simulink model "test_libMdl_Imu"  (R2018a)
settings: Solver=FixedStepAuto  StartTime=0.0  StopTime=50  RelTol=1e-3
libraries: simulink x2, libMdl_Imu x1
settings Model: Creator=hwinter  LastModifiedBy=hwinter

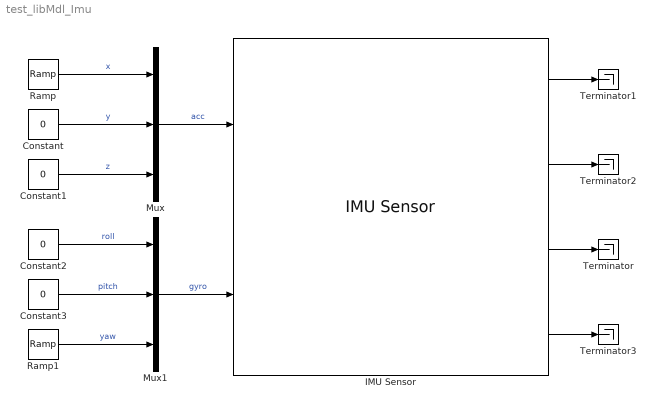
== system test_libMdl_Imu ==
  Constant{,1..3} (4 alike) : Constant  Value=0
  IMU Sensor : libMdl_Imu/IMU Sensor  mv_T_imu=1  mv_sigma_imu_acc=[1 1 1]  mv_sigma_imu_gyro=[1 1 1]  mv_z_0_imu_acc=[0 0 0]  mv_z_0_imu_gyro=[0 0 0]  mv_seed_imu=71322
  Mux : Mux  Inputs=3
  Mux1 : Mux  Inputs=3
  Ramp : simulink/Sources/Ramp  slope=1  start=0  InitialOutput=0
  Ramp1 : simulink/Sources/Ramp  slope=1  start=0  InitialOutput=0
  Terminator{,1..3} (4 alike) : Terminator
  wires:
  Constant/1 -> Mux/2  "y"
  Mux/1 -> IMU Sensor/1  "acc"
  IMU Sensor/3 -> Terminator/1
  IMU Sensor/1 -> Terminator1/1
  Constant1/1 -> Mux/3  "z"
  Mux1/1 -> IMU Sensor/2  "gyro"
  Constant3/1 -> Mux1/2  "pitch"
  Constant2/1 -> Mux1/1  "roll"
  IMU Sensor/4 -> Terminator3/1
  IMU Sensor/2 -> Terminator2/1
  Ramp1/1 -> Mux1/3  "yaw"
  Ramp/1 -> Mux/1  "x"
